simulink model "bus_roadtest_v3"  (R2018a)
settings: Solver=ode3  StartTime=0.0  StopTime=inf  FixedStep=0.01  RelTol=1e-3  EnableMultiTasking=on
PostLoadFcn:
  | , if any(exist('dsrtsu_mdlpostloadfcn', 'file') == [2, 3, 6]), try dsrtsu_mdlpostloadfcn('Execute', bdroot); catch fprintf('Error in PostLoadFcn (dsrtsu_mdlpostloadfcn) for model "%s":\n %s\n', bdroot, lasterr); end, end,
InitFcn:
  | bus_roadtest_v3_initial
values from neighbouring files (symbols this model uses):
  ay_max = 2    [Ini.m]
  delta_t = 0.01    [Ini.m]
  end_left_pass = 1    [Ini.m]
  end_right_pass = 0    [Ini.m]
  finish_node_id = length(Map_data(:,1))    [Ini.m]
  forward_length = 15    [Ini.m]
  gamma = sqrt(N_xaug+lambda)    [bus_roadtest_v3_initial.m]
  k_safe = 1    [Ini.m]
  nodes = nodes(1:index_node,:)    [Ini.m]
  rmin = 10    [Ini.m]
  segments = zeros(length(xy_ends_Pos(:,1)),3)    [Ini.m]
  start_node_id = 1    [Ini.m]
  Ts = 0.01    [bus_roadtest_v3_initial.m]
  Veh_CG = [0.5, 0.2]    [Ini.m]
  Veh_size = [1.99986,6.09558]    [Ini.m]
  vmax = 6    [Ini.m]
  weight = [weight_0,weight_0_cov,weight_i]    [bus_roadtest_v3_initial.m]
undefined symbols (not defined in the file or in its folder): Brake_table, DiscIntNeverNeededParam, Map_data, R, REF_GPS_RFS, Steer_gain_table, T
libraries: rtican x71, simulink x26, rti1401lib_adc_type4 x8, rti1401lib_dio_type4 x1
(part 16 of 18)

== matlab function bus_roadtest_v3/Positioning_module/ITRI_MM/UKF_Only/SLAM_UKF_MM ==
  data: seg_id_near output; Map_data input; dist_op output; Position_X input; op_distance output; Oi_near output; num_lane_direction output; Postion_Y input; Position_H input; seg_heading output; seg_LaneWidth output
function [seg_id_near,dist_op,op_distance,Oi_near,num_lane_direction,seg_heading,seg_LaneWidth]= fcn(Map_data,Position_X,Postion_Y,Position_H)

%%% Map_data=[Seg_XY SLOPE_SEG SHIFT_SEG Heading_X LENGTH_SEG]; nx8
XY_ID=Map_data(:,1);
XY_INI=Map_data(:,2:3);
XY_END=Map_data(:,4:5);
SLOPE_SEG=Map_data(:,6);
SHIFT_SEG=Map_data(:,7);
HEADING_DIFFERENCE_VEH_ROAD = 45*pi/180;
DIST_THREAD_5 = 4;

m=length(XY_ID);
oi_xy=zeros(m,2);
dist_op=zeros(m,1);
for i =1:m
    if SLOPE_SEG(i) == inf
        oi_xy(i,1) = XY_INI(i,1); % x position of the projection point on this segment
        oi_xy(i,2) = Postion_Y;
    elseif SLOPE_SEG(i)==0
        oi_xy(i,1) = Position_X;
        oi_xy(i,2) = XY_INI(i,2);
    else
        a_j = -1/SLOPE_SEG(i);
        b_j = Postion_Y - a_j*Position_X;
        oi_xy(i,1) = (b_j-SHIFT_SEG(i))/(SLOPE_SEG(i)-a_j); % x position of the i-th projection point
        oi_xy(i,2) = (SLOPE_SEG(i)*b_j - a_j*SHIFT_SEG(i))/(SLOPE_SEG(i)-a_j); % y position of the i-th projection point 
    end          
end

for i = 1:length(oi_xy(:,1))
    dist_op(i,1)=sqrt((oi_xy(i,1)-Position_X)^2+(oi_xy(i,2)-Postion_Y)^2);     
end

[seg_id_near,op_distance,oi_near,note,seg_direction,head_err,num_lane_direction,seg_heading] = MM(Position_H*180/pi,[Position_X;Postion_Y],oi_xy,dist_op,Map_data,HEADING_DIFFERENCE_VEH_ROAD,DIST_THREAD_5);
Oi_near=oi_near';
[~,seg_id_ind] = max(XY_ID == seg_id_near);
seg_LaneWidth = Map_data(seg_id_ind,11);
seg_Curvature = Map_data(seg_id_ind,14);

%% MM function
function [seg_id_near,op_distance,oi_near,note,seg_direction,head_err,num_lane_direction,seg_heading] = MM(heading,X_pos,oi_xy,dist_op,Map_data,HEADING_DIFFERENCE_VEH_ROAD,DIST_THREAD_5)
note=0;
seg_id_near=double(0);
op_distance=0;
oi_near=zeros(1,2);
end_pt=zeros(1,2);
seg_direction=0;
[dist_sort,index] = sort(dist_op);
index=[index,zeros(length(index),1)];

xy_ini = Map_data(:,2:3);
xy_end = Map_data(:,4:5);
SLOPE_SEG = Map_data(:,6);
seg_id = Map_data(:,1);
LENGTH_SEG = Map_data(:,9);
SEG_GPS_HEAD = Map_data(:,8);
SEG_GPS_HEAD=[seg_id SEG_GPS_HEAD];

%%    Map Matching

for j = 1:length(xy_ini(:,1));
    i = index(j,1);
    dis_temp1 = sqrt((xy_ini(i,1)-oi_xy(i,1))^2+(xy_ini(i,2)-oi_xy(i,2))^2);
    dis_temp2 = sqrt((xy_end(i,1)-oi_xy(i,1))^2+(xy_end(i,2)-oi_xy(i,2))^2);
 
    if (dis_temp1 <= LENGTH_SEG(i)&& dis_temp2 <= LENGTH_SEG(i));
        index(j,2) = 1; %oi_xy lies in between xy_ini and xy_end
    else index(j,2) = 0;
    end
end

%"possible_seg" contains the sequence of possible segment index
ind_temp = find(index(1:end,2)==1);
% ind_temp=ind_temp(1);
if isempty(ind_temp);
   note = 1;  % 1: the projection point is not between two segment ends for any road segment;
              % search nearest segment by finding the nearest segment end!             
   %compare distances between ends and X_pos!     
    dist_ini = rel_dist_xy(X_pos,xy_ini);
    dist_end = rel_dist_xy(X_pos,xy_end);
  
    [min_dis_ini,junk1] = min(dist_ini);   %-------------------------------------------------哪來的junk 1 &2 ?
    [min_dis_end,junk2] = min(dist_end);
    if min_dis_ini<= min_dis_end; %X_pos is closer to the end
       possible_seg = junk1; %index
       end_pt = xy_ini(junk1,1:end);
    else 
       possible_seg = junk2; %index
       end_pt = xy_end(junk2,1:end);
    end

    seg_id_near = seg_id(possible_seg);
    
    op_distance = dist_op(possible_seg);
    oi_near = oi_xy(possible_seg,1:2);
    if possible_seg>1 && possible_seg<length(seg_id)
    op_distance_n=rel_dist_xy(X_pos,oi_near);
    min_ini_pos=rel_dist_xy(X_pos,xy_ini(possible_seg,:));
    min_end_pos=rel_dist_xy(X_pos,xy_end(possible_seg,:));
    if op_distance_n<min_ini_pos && op_distance_n<min_end_pos
        note = 0;
    else
        note = 1;
    end
    else
        op_distance_n=rel_dist_xy(X_pos,oi_near);
        min_ini_pos=rel_dist_xy(X_pos,xy_ini(possible_seg,:));
        min_end_pos=rel_dist_xy(X_pos,xy_end(possible_seg,:));
    end
    
%    seg_direction = Get_Seg_Heading(seg_id_near,heading);
%    %%%不用老師程式--
    [~,temp_ind] = max(SEG_GPS_HEAD(:,1) == seg_id_near);
    head_err = abs(heading-SEG_GPS_HEAD(temp_ind(1),2)); 
    if head_err <= HEADING_DIFFERENCE_VEH_ROAD
    seg_direction = 1; %1= along slope, 2:adverse
    elseif head_err>=HEADING_DIFFERENCE_VEH_ROAD && head_err<=90
    seg_direction = 0; %unknown
    else
    seg_direction = 2;
    end
%     %%%不用老師程式--
 elseif length(ind_temp(1)) ==1; %only 
%      find one segment candidate
       note = 0; % 0: the projection point lies between two ends of each segment    
       possible_seg = index(ind_temp(1),1);
       seg_id_near = seg_id(possible_seg);
       op_distance = dist_op(possible_seg);
       oi_near = oi_xy(possible_seg,1:2);
       end_pt = [0,0]; % temp./unused nominal values
%      seg_direction = Get_Seg_Heading(seg_id_near,heading); %get road segment heading direction

        [~,temp_ind] = max(SEG_GPS_HEAD(:,1) == seg_id_near);
        head_err = abs(heading-SEG_GPS_HEAD(temp_ind(1),2)); 
       if head_err <= HEADING_DIFFERENCE_VEH_ROAD;
            seg_direction = 1; %1= along slope, 2:adverse
       elseif head_err>=HEADING_DIFFERENCE_VEH_ROAD && head_err<=90
            seg_direction = 0; %unknown
       else
            seg_direction = 2;
       end
       %Now compare the distances between X_pos and all segment ends with
       %op_distance. If find closer node, may discard previous found segment.
       
       dist_ini = rel_dist_xy(X_pos,xy_ini);
       dist_end = rel_dist_xy(X_pos,xy_end);
           %dis_min = min(dist_ini,dist_end);
           %dis_min_val = min(dis_min);
           %temp_a = find(dis_min == dis_min_val); % diff, segments may have the same node!
       [min_dis_ini,junk1] = min(dist_ini);
       [min_dis_end,junk2] = min(dist_end);
       dis_min_val = min(min_dis_ini,min_dis_end);
       
    if dis_min_val < op_distance;%min(op_distance); %X_pos is closer to one of the segment ends than its project point         
       note = 2; %Change the "note" value! 
                 %special case: the found projection pt. (oi_near) lie(s) between two ends 
                 %of one segment, but the associated segments may not
                 %the nearest road segments.          
       %search the nearest node of road segments. 
        if min_dis_ini<= min_dis_end;
           temp_a = junk1;
           end_pt = xy_ini(junk1,1:end);
        else 
           temp_a = junk2;
           end_pt = xy_end(junk2,1:end);
        end
       
        
        if length(temp_a)>1; %multiple segment case
            
           seg_head_pos = SEG_GPS_HEAD(temp_a,2); %road segment heading in the positive slope direction
%            seg_head_neg = SEG_GPS_HEAD(temp_a,3);
           
           %find smallest heading discrepancy in positive slope direction
           [junk1,ind_pos] = min(abs(heading - seg_head_pos(1:end)));
               
           %find smallest heading discrepancy in negative/adverse slope direction
%            [junk2,ind_neg] = min(abs(angle_convert(heading - seg_head_neg(1:end))));
           
           %compare two smallest heading erros of two adverse directions
 
              ind = temp_a(ind_pos);
              seg_id_near = seg_id(ind);
              op_distance = dist_op(ind);
              oi_near = oi_xy(ind,1:2);
              [~,temp_ind] = max(SEG_GPS_HEAD(:,1) == seg_id_near);
              head_err = abs(heading-SEG_GPS_HEAD(temp_ind(1),2)); 

              if head_err <= HEADING_DIFFERENCE_VEH_ROAD;
                    seg_direction = 1; %1= along slope, 2:adverse
              elseif head_err>=HEADING_DIFFERENCE_VEH_ROAD && head_err<=90
                    seg_direction = 0; %unknown
              else
                    seg_direction = 2;
              end
       
        else %single segment case
              [~,temp_ind] = max(SEG_GPS_HEAD(:,1) == seg_id_near);
              head_err = abs(heading-SEG_GPS_HEAD(temp_ind(1),2)); 

              if head_err <= HEADING_DIFFERENCE_VEH_ROAD;
                    seg_direction = 1; %1= along slope, 2:adverse
              elseif head_err>=HEADING_DIFFERENCE_VEH_ROAD && head_err<=90
                    seg_direction = 0; %unknown
              else
                    seg_direction = 2;
              end
                 seg_id_near = seg_id(temp_a);
                 op_distance = dist_op(temp_a);
                 oi_near = oi_xy(temp_a,1:2);
        end
    end
 else %multiple segment candidates
       note = 0; % 0: the projection point lies between two ends of each segment          
       cand_seg = index(ind_temp(1),1);
       %cand_id = seg_id(cand_seg(1:2)); % only check the first two colsest segment candidate
       cand_op_dist = dist_op(cand_seg(1:2));
       
       %find road heading for the first two candidates
        head_pos = SEG_GPS_HEAD(cand_seg(1:2),2);

       %first candidate
        err_1 =  abs(heading - head_pos(1));
        %temp = [head_pos(1),head_neg(1)];
        %cand_head(1) = temp(ii);
        %clear ii;
       %second candidate
        err_2 = abs(heading - head_pos(2));
        %temp = [head_pos(2),head_neg(2)];
        %cand_head(2) = temp(ii);
        %clear ii;
        
       %compare two heading errors
        if err_1<= err_2 && err_1< HEADING_DIFFERENCE_VEH_ROAD; % HEADING_DIFFERENCE_VEH_ROAD = 45/180*pi
           possible_seg =  cand_seg(1);
           seg_direction = 1;
        elseif err_2< err_1 && ((cand_op_dist(2)-cand_op_dist(1))< DIST_THREAD_5); %DIST_THREAD_5 = 9 m
           possible_seg = cand_seg(2); 
           seg_direction = 2;
        else
           possible_seg = cand_seg(1);
           seg_direction = 1;
        end
        
       clear err_1 err_2 cand_op_dist cand_seg head_pos head_neg direction_1 direction_2;
       %possible_seg = index(ind_temp,1);       
       seg_id_near = seg_id(possible_seg);
       op_distance = dist_op(possible_seg);
       oi_near = oi_xy(possible_seg,1:2);
       end_pt = [0,0]; % temp./unused nominal values
        
       %Now compare the distances between X_pos and all segment ends with
       %above op_distance.
       %compute distances between X_pos and all segment ends
       dist_ini = rel_dist_xy(X_pos,xy_ini);
       dist_end = rel_dist_xy(X_pos,xy_end);
           %dis_min = min(dist_ini,dist_end);
           %dis_min_val = min(dis_min);
           %temp_a = find(dis_min == dis_min_val); % diff, segments may have the same node!
       [min_dis_ini,junk1] = min(dist_ini);
       [min_dis_end,junk2] = min(dist_end);
       dis_min_val = min(min_dis_ini,min_dis_end); 
       
    if dis_min_val < op_distance; %min(op_distance); %X_pos is closer to one of the segment ends than its project point         
       note = 2; %Change the note value! 
                 %special case: the found projection pt. (oi_near) lie(s) between two ends 
                 %of one segment, but the associated segments may not be
                 %the nearest road segments.          
       %search the nearest node of road segments. 
        if min_dis_ini<= min_dis_end;
           temp_a = junk1;
           end_pt = xy_ini(junk1,1:2);
        else 
           temp_a = junk2;
           end_pt = xy_end(junk2,1:2);
        end
        clear junk1 junk2;
        
        if length(temp_a)>1; %multiple segment case, then compare heading with road segment heading
          
           seg_head_pos = SEG_GPS_HEAD(temp_a,2);
           [junk1,ind_pos] = min(abs(heading - seg_head_pos(1:end)));


              ind = temp_a(ind_pos);
              seg_id_near = seg_id(ind);
              op_distance = dist_op(ind);
              oi_near = oi_xy(ind,1:2);

              [~,temp_ind] = max(SEG_GPS_HEAD(:,1) == seg_id_near);
              head_err = abs(heading-SEG_GPS_HEAD(temp_ind(1),2)); 

              if head_err <= HEADING_DIFFERENCE_VEH_ROAD;
                    seg_direction = 1; %1= along slope, 2:adverse
              elseif head_err>=HEADING_DIFFERENCE_VEH_ROAD && head_err<=90
                    seg_direction = 0; %unknown
              else
                    seg_direction = 2;
              end

       
        else %determine road direction is positive or negative slope direction

             seg_id_near = seg_id(temp_a);
             op_distance = dist_op(temp_a);
             oi_near = oi_xy(temp_a,1:2);
             [~,temp_ind] = max(SEG_GPS_HEAD(:,1) == seg_id_near);
              head_err = abs(heading-SEG_GPS_HEAD(temp_ind(1),2)); 

              if head_err <= HEADING_DIFFERENCE_VEH_ROAD;
                    seg_direction = 1; %1= along slope, 2:adverse
              elseif head_err>=HEADING_DIFFERENCE_VEH_ROAD && head_err<=90
                    seg_direction = 0; %unknown
              else
                    seg_direction = 2;
              end

        end
    end
           
end
%% check projection distance positive or negative Y=AX+B ;AX+B-Y>0 or AX+B-Y<0
Heading_X_rad = Map_data(:,8).*pi./180;
[~,temp_ind] = max(seg_id(:,1) == seg_id_near);
A=SLOPE_SEG(temp_ind);
B=oi_near(2)-A*oi_near(1);
if A < 0
    C=-A*X_pos(1)-B+X_pos(2);
    if Heading_X_rad(temp_ind) > 3*pi/2 && Heading_X_rad(temp_ind) < 2*pi
        C = C;
    else
        C = -C;
    end
elseif A == 0
    if oi_near(2)<X_pos(2)
        C=-1;
    else
        C=1;
    end
else
    C=A*X_pos(1)+B-X_pos(2);
    if Heading_X_rad(temp_ind) > pi && Heading_X_rad(temp_ind) < 3*pi/2
        C = C;
    else
        C = -C;
    end
end
if C<0 
    d=1;
elseif C==0
    d=1;
else
    d=-1;
end
num_lane_direction=[A;B;C;d];
seg_heading = Heading_X_rad(temp_ind);
%% rel_dist
function dist = rel_dist_xy(ref_xy,pt_xy)
% This function computes relative distances between given reference point, ref_xy, and positions, p_xy. 
% ref_xy = [x0,y0];
% pt_xy = [x,y];

temp = (pt_xy(:,1)-ref_xy(1)).^2 + (pt_xy(:,2)-ref_xy(2)).^2;
dist = temp.^0.5;

== matlab function bus_roadtest_v3/Positioning_module/ITRI_MM/UKF_Only/SLAM_UKF ==
  data: Q input; R input; X output; X_AUG input; X_state input; IMU_Sensor input; Sensor_dt input; SLAM_update input; weighting input; P output; K output; x_aug output; d_GC input
function [X,P,K,x_aug] = fcn(Q,R,X_AUG,X_state,IMU_Sensor,Sensor_dt,SLAM_update,weighting,d_GC)
%#codegen

%% parameters setup

%%% X_State=[X,Y,Heading]
x_aug=X_AUG(:,1:11);
vx=IMU_Sensor(1)*1;
wz=IMU_Sensor(2);
Grade=IMU_Sensor(3);
dt=Sensor_dt;
weight_0=weighting(1);
weight_0_cov=weighting(2);
weight_i=weighting(3);
X=zeros(5,1);
N=5;

%%
%%% model 1 : slope detection
    x_aug(1,:) = x_aug(1,:) + (dt*x_aug(5,:)).*cos(x_aug(3,:)) + dt.*wz*d_GC*cos(x_aug(3,:)+pi/2); %north
    x_aug(2,:) = x_aug(2,:) + (dt*x_aug(5,:)).*sin(x_aug(3,:)) + dt.*wz*d_GC*sin(x_aug(3,:)+pi/2);%east
    x_aug(3,:) = x_aug(3,:) + (dt.*x_aug(4,:));                  %heading (radian)
    x_aug(4,:) = x_aug(4,:);
    x_aug(5,:) = x_aug(5,:);
    

 %% state process

X(1,1) = x_aug(1,1)*weight_0 + sum(x_aug(1,2:end))*weight_i;
X(2,1) = x_aug(2,1)*weight_0 + sum(x_aug(2,2:end))*weight_i;
X(3,1) = x_aug(3,1)*weight_0 + sum(x_aug(3,2:end))*weight_i;
X(4,1) = x_aug(4,1)*weight_0 + sum(x_aug(4,2:end))*weight_i;
X(5,1) = x_aug(5,1)*weight_0 + sum(x_aug(5,2:end))*weight_i;
% X = X*10^6;

    P = weight_0_cov.*((x_aug(1:5,1)-X(1:5,1))*(x_aug(1:5,1)-X(1:5,1))');

for i = 2:(2*N+1)
    
    P = P + weight_i.*((x_aug(1:5,i)-X(1:5,1))*(x_aug(1:5,i)-X(1:5,1))');

end
% P = P*10^6;

P = P + Q;

if X(3,1) < 0
    X(3,1) = X(3,1) + 2*pi;
elseif X(3,1) >= 2*pi
    X(3,1) = X(3,1) - 2*pi;
else
    X(3,1) = X(3,1);
end
%% kalman filter
if SLAM_update >0 %close-loop
    
 
        Z = X_state;

        Z_e = X; %=H*X; % observation estimate using a-priori state estimate
   %K = P*H'*inv(H*P*H'+R); % Kalman gain
        K = P*inv(P+R); %H = eye(3) %K = P*inv(P+R)
   %X = X + K*(Z - Z_e); % a-posteriori state estimate
        dZ = Z - Z_e;
        X = X + K*dZ; % a-posteriori state estimate
   
   %P = (eye(3) - K*H)*P;
  
   
        P = (eye(5) - K)*P;

        
else %open loop
        
        K = zeros(5,5);
        Z = X_state([4,5]); 
        Z_e = X([4,5]); %=H*X; % observation estimate using a-priori state estimate
   %K = P*H'*inv(H*P*H'+R); % Kalman gain
        K1 = P([4,5],([4,5]))*inv(P([4,5],([4,5]))+R([4,5],([4,5]))); %H = eye(3)
   %X = X + K*(Z - Z_e); % a-posteriori state estimate
        dZ = Z - Z_e;
        X([4,5]) = X([4,5]) + K1*dZ; % a-posteriori state estimate
   
   %P = (eye(3) - K*H)*P;
    
        P([4,5],([4,5])) = (eye(2) - K1)*P([4,5],([4,5]));
end


function dist = rel_dist_xy(ref_xy,pt_xy)
% This function computes relative distances between given reference point, ref_xy, and positions, p_xy. 
% ref_xy = [x0,y0];
% pt_xy = [x,y];

temp = (pt_xy(:,1)-ref_xy(1)).^2 + (pt_xy(:,2)-ref_xy(2)).^2;
dist = temp.^0.5;

== matlab function bus_roadtest_v3/Positioning_module/ITRI_MM/UKF_Only/SLAM_Check ==
  data: SLAM_fault input; SLAM_X input; SLAM_update output; SLAM_Y input; SLAM_Heading input; SLAM_Counter input; IMU_Sensor input; X_UKF input; SLAM_FS input; Q_last_i input; R_last_i input; Last_SLAM_In input; X_state output; SLAM_FaultFlag output; Q_last_o output; R_last_o output; Last_SLAM_Out output; count_i input; count_o output; dist_SLAMlastUKFSLAM output; SLAM_FaultFlag_case output
function [SLAM_update,X_state,SLAM_FaultFlag,Q_last_o,R_last_o,Last_SLAM_Out,count_o,dist_SLAMlastUKFSLAM,SLAM_FaultFlag_case] = fcn(SLAM_fault,SLAM_X,SLAM_Y,SLAM_Heading,SLAM_Counter,IMU_Sensor,X_UKF,SLAM_FS,Q_last_i,R_last_i,Last_SLAM_In,count_i)

Last_X=Last_SLAM_In(1);
Last_Y=Last_SLAM_In(2);
Last_Heading = Last_SLAM_In(3);
Last_Counter = Last_SLAM_In(4);

Sensor_Velocity = IMU_Sensor(1);
Sensor_Yawrate=IMU_Sensor(2);
Sensor_Grade=IMU_Sensor(3);

SLAM_FaultFlag = 0;
SLAM_update = 0;

if SLAM_Counter ~= Last_Counter
    SLAM_update = 1;
    count_o = 0;
else
    count_o = count_i + 1;
end

if SLAM_fault == 1
    SLAM_update = 0;
end

SLAM_FaultFlag_case = 0;
dist_SLAMlastUKFSLAM = sqrt((SLAM_X-X_UKF(1))^2 + (SLAM_Y-X_UKF(2))^2); %跟上一刻估測值差異
dist_SLAMlastSLAM =  sqrt((SLAM_X-Last_X)^2 + (SLAM_Y-Last_Y)^2); %跟上一刻量測值差異
Heading_diff = abs(SLAM_Heading-Last_Heading);
if Heading_diff > pi
    Heading_diff = 2*pi - Heading_diff;
end
if Sensor_Velocity < 0.01
    if SLAM_fault == 1 || count_o > 100 || dist_SLAMlastUKFSLAM > 0.1
        SLAM_FaultFlag = 1;
        SLAM_FaultFlag_case = 1;
    end
    if SLAM_update > 0 && dist_SLAMlastSLAM > 0.1
        SLAM_FaultFlag = 1;
        SLAM_FaultFlag_case = 2;
    end
    if SLAM_update > 0 && Heading_diff > 20*pi/180
        SLAM_FaultFlag = 1;
        SLAM_FaultFlag_case = 3;
    end
else
    if SLAM_fault == 1 || count_o > 200 || dist_SLAMlastUKFSLAM > 5
        SLAM_FaultFlag = 1;
        SLAM_FaultFlag_case = 4;
    end
end

if abs(SLAM_Heading - X_UKF(3)) > 5.5
    H_ACC = 100;
else
    H_ACC = 0.1;
end

if SLAM_update == 0
    SLAM_X_out = Last_X;
    SLAM_Y_out = Last_Y;
    SLAM_Heading_out = Last_Heading;
    Q = Q_last_i;
    R = R_last_i;
else
    SLAM_X_out = SLAM_X;
    SLAM_Y_out = SLAM_Y;
    SLAM_Heading_out = SLAM_Heading;
    Q = diag([0.00025,0.00025,0.0000001,0.00001,0.0001]);
    R = diag([(0.01)^2,(0.01)^2,H_ACC,0.1,0.0001]);
end

Q_last_o = Q;
R_last_o = R;
SLAM_Counter_out = SLAM_Counter;

Last_SLAM_Out = [SLAM_X_out;SLAM_Y_out;SLAM_Heading_out;SLAM_Counter_out];
X_state = [SLAM_X_out,SLAM_Y_out,SLAM_Heading_out,Sensor_Yawrate,Sensor_Velocity]';

== matlab function bus_roadtest_v3/Speed_profile/Auto & Check/Auto_Door ==
  settings: updateMethod=DISCRETE
  data: Static_flag input; Auto_Door output; Stop_Check input; Door_count output
function [Auto_Door, Door_count] = fcn(Static_flag,Stop_Check)
persistent counting Stop_state
if isempty(counting)
    counting = 0;
    Stop_state = 0;
end
Auto_Door = 0;

if Stop_Check ==1
    Stop_state = 1;
end
if Stop_state==1 && Static_flag==1
    counting = counting+1;
end
if counting>300
    Auto_Door=1;
    Stop_state = 0;
    counting = 0;
end
Door_count = counting;

== matlab function bus_roadtest_v3/Data_RX/X-by-wire/Steer/CAN_timeout_checker ==
  data: RX_sig input; timeout output
function timeout = fcn(RX_sig)
persistent counter
if isempty(counter)
    counter = 0;
end

if (RX_sig == 0)
    counter = counter +1;
else
    counter = 0;
end

if counter >= 80
    timeout = 1;
else
    timeout = 0;
end

== matlab function bus_roadtest_v3/Target_planner/Path_Output ==
  settings: updateMethod=DISCRETE  sampleTime=0.01
  data: Vehicle_state input; Path_LV output; Path_x input; Path_y input
function Path_LV  = TargetDecision(Vehicle_state,Path_x,Path_y)
%% projection Path to LiDAR view
x = Vehicle_state(1,1);
y = Vehicle_state(2,1);
heading = Vehicle_state(3,1);

Path_LV = zeros(2,6);
% for i =1:6
%     j = i + 1;
%     rotate_ang_path = (heading-pi/2);
%     Path_LV(1:2,i) = [cos(rotate_ang_path),sin(rotate_ang_path);-sin(rotate_ang_path),cos(rotate_ang_path)]*[Path_x(j)-x;Path_y(j)-y];
% end

== matlab function bus_roadtest_v3/Flag_management/Fault detection/Fault detection(Control)/Brake fault detection/MATLAB Function2 ==
  data: u input; y output
function y = my_average(u) %# codegen
persistent i buf bufSum;
if isempty(buf)
    buf = zeros(1,300); %averaging steps
    bufSum = 0;
    i = 1;
end
bufSum = bufSum - buf(i);
buf(i) = u;
bufSum = bufSum + u;
i = i + 1;
if i > numel(buf)
    i = 1;
end
y = bufSum / numel(buf);

== matlab function bus_roadtest_v3/Flag_management/Fault detection/Fault detection(Control)/Steer fault detection/MATLAB Function4 ==
  settings: updateMethod=DISCRETE
  data: u input; y output
function y = my_average(u) %# codegen
persistent i buf bufSum;
if isempty(buf)
    buf = zeros(1,200); %averaging steps
    bufSum = 0;
    i = 1;
end
bufSum = bufSum - buf(i);
buf(i) = u;
bufSum = bufSum + u;
i = i + 1;
if i > numel(buf)
    i = 1;
end
y = bufSum / numel(buf);

== matlab function bus_roadtest_v3/Flag_management/Fault detection/Fault detection(Control)/Steer fault detection/MATLAB Function5 ==
  settings: updateMethod=DISCRETE
  data: u input; y output
function y = my_average(u) %# codegen
persistent i buf bufSum;
if isempty(buf)
    buf = zeros(1,50); %averaging steps
    bufSum = 0;
    i = 1;
end
bufSum = bufSum - buf(i);
buf(i) = u;
bufSum = bufSum + u;
i = i + 1;
if i > numel(buf)
    i = 1;
end
y = bufSum / numel(buf);

== matlab function bus_roadtest_v3/Flag_management/Fault detection/Fault detection(Control)/Speed fault detection/MATLAB Function6 ==
  settings: updateMethod=DISCRETE
  data: u input; y output
function y = my_average(u) %# codegen
persistent i buf bufSum;
if isempty(buf)
    buf = zeros(1,500); %averaging steps
    bufSum = 0;
    i = 1;
end
bufSum = bufSum - buf(i);
buf(i) = u;
bufSum = bufSum + u;
i = i + 1;
if i > numel(buf)
    i = 1;
end
y = bufSum / numel(buf);

== matlab function bus_roadtest_v3/Flag_management/Fault detection/Fault detection(Control)/Speed fault detection/MATLAB Function7 ==
  settings: updateMethod=DISCRETE
  data: u input; y output
function y = my_average(u) %# codegen
persistent i buf bufSum;
if isempty(buf)
    buf = zeros(1,50); %averaging steps
    bufSum = 0;
    i = 1;
end
bufSum = bufSum - buf(i);
buf(i) = u;
bufSum = bufSum + u;
i = i + 1;
if i > numel(buf)
    i = 1;
end
y = bufSum / numel(buf);

== matlab function bus_roadtest_v3/Flag_management/Fault detection/Fault detection(Control)/OBU fault detection ==
  data: SPAT input; OBU_fault output; counting output
function [OBU_fault, counting] = fcn(SPAT)

persistent count;
if isempty(count)
    count = 0;
end

count = count +1;
if SPAT == 1
    count = 0;
end
OBU_fault = 0;
if count>300
    OBU_fault = 1;
end
counting = count;

== matlab function bus_roadtest_v3/Flag_management/Fault detection/Fault flags management ==
  data: Fault_minor output; Fault_prime output; Monitor_fault input; OBU_fault input; Speed_fault input; Steer_fault input; Brake_fault input; RSU_fault input; SLAM_fault input
function [Fault_minor, Fault_prime] = fcn(Monitor_fault, OBU_fault, Speed_fault, Steer_fault, Brake_fault,RSU_fault,SLAM_fault)
Fault_prime = max([Monitor_fault, OBU_fault, Speed_fault, Steer_fault, Brake_fault, RSU_fault, SLAM_fault]);
% if Uturn_flag==1
%     Fault_prime = 0;
% end
Fault_minor = 0;

== matlab function bus_roadtest_v3/Flag_management/Button management/Button management ==
  settings: updateMethod=DISCRETE
  data: Drive_start_button input; Drive_stop_button input; Drive_start output; Emergency_button input; Door_state_fb input; Door1_open_button input; Door1_close_button input; Door2_button input; Door_switch_button input; Drive_stop output; Emergency_stop output; Door_cmd output; Auto_Door input
function [Drive_start, Drive_stop, Emergency_stop, Door_cmd] = Button_management(Drive_start_button, Drive_stop_button, Emergency_button, Door_state_fb, Door1_open_button, Door1_close_button, Door2_button, Door_switch_button, Auto_Door)

%For Door control
% Door_switch   0=Operator  1=Passenger
% Door_state    0 = close   1 = open  
%Door_button = [Door_state_fb, Door1_open_button, Door1_close_button, Door2_button, Door_switch_button];

persistent Door_state Time_count;
if isempty(Time_count)
    Door_state = Door_state_fb;
    Time_count = 0;
end 

if Door_switch_button == 0
    if Door1_open_button ==1
        Door_state = 1;
    elseif Door1_close_button ==1
        Door_state = 0;
    end
elseif Door_switch_button == 1
    if  Door2_button ==1 && Time_count >500  % Door can't change twice within 5 second
        if Door_state ==1
            Door_state = 0;
        else
            Door_state = 1;
        end
        Time_count = 0;
    end
    if Door1_open_button ==1
        Door_state = 1;
    elseif Door1_close_button ==1
        Door_state = 0;
    end
end
Time_count = Time_count + 1;
if Auto_Door ==1
    Door_state = 1;
end



Door_cmd = Door_state;
Emergency_stop = Emergency_button; 
Drive_start =Drive_start_button;
Drive_stop = Drive_stop_button;




%%%%%%%%%%%%%%%%%%%%%%%%%%%%%%%%%%%%%%%%%%%%%%%%%%%%%%%%%%%%%%%%%%%%%%%%%%%

== matlab function bus_roadtest_v3/Data_RX/X-by-wire/Brake/CAN_timeout_checker ==
  data: RX_sig input; timeout output
function timeout = fcn(RX_sig)
persistent counter
if isempty(counter)
    counter = 0;
end

if (RX_sig == 0)
    counter = counter +1;
else
    counter = 0;
end

if counter >= 80
    timeout = 1;
else
    timeout = 0;
end

== matlab function bus_roadtest_v3/Data_RX/Control_button/MATLAB Function2 ==
  settings: updateMethod=DISCRETE
  data: u input; y output; yy output
function [y,yy]= fcn(u)
%#codegen
persistent y2 y1 ;
if isempty(y2)
    y2 = 0;
    y1 = 0;
end 
if u ==1
    y2 = 1;
end
yy = y2;
y = y1;

== matlab function bus_roadtest_v3/Data_RX/X-by-wire/Brake/CAN_timeout_checker1 ==
  data: RX_sig input; timeout output
function timeout = fcn(RX_sig)
persistent counter
if isempty(counter)
    counter = 0;
end

if (RX_sig == 0)
    counter = counter +1;
else
    counter = 0;
end

if counter >= 80
    timeout = 1;
else
    timeout = 0;
end

== matlab function bus_roadtest_v3/Data_RX/X-by-wire/Throttle/CAN_timeout_checker ==
  data: RX_sig input; timeout output
function timeout = fcn(RX_sig)
persistent counter
if isempty(counter)
    counter = 0;
end

if (RX_sig == 0)
    counter = counter +1;
else
    counter = 0;
end

if counter >= 80
    timeout = 1;
else
    timeout = 0;
end

== matlab function bus_roadtest_v3/Data_RX/OBU/Light_state_DSRC ==
  settings: updateMethod=DISCRETE
  data: SLAM_seg_id_near input; phase_01 input; Light_info_out output; phase_02 input; phase_03 input; phase_04 input; phase_05 input; phase_06 input; phase_07 input; phase_08 input; RT_01 input; RT_02 input; RT_03 input; RT_04 input; RT_05 input; red output; left output; last_phase input
function [Light_info_out,red,left]     = fcn(SLAM_seg_id_near,phase_01,phase_02,phase_03,phase_04,phase_05,phase_06,phase_07,phase_08, RT_01, RT_02, RT_03, RT_04,RT_05,last_phase)

% output light info 0=no message, 1=red, 2=green,3=yellow

persistent Light_info;
if isempty(Light_info)
    Light_info = 0;
end 
phase01 = de2bi(phase_01);
phase02 = de2bi(phase_02);
if phase_02<128
    phase02(8)=0;
end
phase03 = de2bi(phase_03);
phase04 = de2bi(phase_04);
phase05 = de2bi(phase_05);
phase06 = de2bi(phase_06);
phase07 = de2bi(phase_07);
phase08 = de2bi(phase_08);

if SLAM_seg_id_near>=999 && SLAM_seg_id_near<134
    if phase01(6)==1  || phase01(4)==1
        Light_info =2;
    else
        Light_info =1;
    end
% elseif SLAM_seg_id_near>=134 && SLAM_seg_id_near<154
% || (phase02(8)==1&&last_phase==0&&RT_02<10)
elseif SLAM_seg_id_near>=134 && SLAM_seg_id_near<154
     if (phase02(6)==1&&RT_02>2)  || (phase02(5)==1&&RT_02>2) || (phase02(8)==1&&last_phase==0&&RT_02<16)
        Light_info =2;
    else
        Light_info =1;
    end
elseif SLAM_seg_id_near>=218 && SLAM_seg_id_near<238
    if (phase05(6)==1&&RT_05>3)  || phase05(4)==1
        Light_info =2;
    else
        Light_info =1;
    end
elseif SLAM_seg_id_near>=238 && SLAM_seg_id_near<252
    if (phase04(6)==1&&RT_04>3)  || phase04(4)==1
        Light_info =2;
    else
        Light_info =1;
    end
elseif SLAM_seg_id_near>=252 && SLAM_seg_id_near<267
    if (phase03(6)==1&&RT_03>3)  || phase03(5)==1
        Light_info =2;
    else
        Light_info =1;
    end
elseif SLAM_seg_id_near>=309 && SLAM_seg_id_near<329
    if phase08(6)==1  || phase08(5)==1
        Light_info =2;
    else
        Light_info =1;
    end
else
    Light_info =0;
end

Light_info_out = Light_info;
red = phase02(8);
left = phase02(5);

== matlab function bus_roadtest_v3/Data_RX/X-by-wire/Input_speed/MATLAB Function ==
  settings: updateMethod=DISCRETE
  data: Speed_raw input; Speed_mps output; Rate_limit input
function Speed_mps = Spike_filter(Speed_raw,Rate_limit)

persistent Speed_mps_last
if isempty(Speed_mps_last)
    Speed_mps_last = 0;
end 

if abs(Speed_raw - Speed_mps_last) > Rate_limit
    Speed_mps = Speed_mps_last + sign(Speed_raw-Speed_mps_last) * Rate_limit;
else
    Speed_mps = Speed_raw;
end

Speed_mps_last = Speed_mps;

== matlab function bus_roadtest_v3/Data_RX/Xavier/Filter1/MATLAB Function ==
  data: GF input; GF_filtered output; GF_last input
function GF_filtered  = fcn(GF,GF_last)
persistent count
if isempty(count)
    count = 0;
end

if (GF_last-GF) > 200 && count<20
    GF_filtered = GF_last;
    count = count+1;
else
    GF_filtered = GF;
    count = 0;
end

== matlab function bus_roadtest_v3/Data_RX/Xavier/Filter2/MATLAB Function ==
  data: GF input; GF_filtered output; GF_last input
function GF_filtered  = fcn(GF,GF_last)
persistent count
if isempty(count)
    count = 0;
end

if (GF_last-GF) > 200 && count<10
    GF_filtered = GF_last;
    count = count+1;
else
    GF_filtered = GF;
    count = 0;
end

== matlab function bus_roadtest_v3/Data_RX/OBU/Check_New_SBG_and_x_y_coordination ==
  data: x output; y output; SBG_long input; SBG_lat input; SBG_alt input; REF_GPS_RFS input; z output
function [x,y,z] = fcn(SBG_long,SBG_lat,SBG_alt,REF_GPS_RFS)
%#codegen
[x,y,z] = dllh2denu(REF_GPS_RFS,[SBG_long,SBG_lat,SBG_alt]) ;

function [de,dn,du] =dllh2denu(llh0,llh)
%%% approximation version for GPS coordinate transformation from
%%% llh(longitude,latitude,altitude) to [de,dn,du]=(east,north,height) relatitive to a
%%% given reference point,llh0
% REF_GPS_RFS = [122.000000+20.0304416/60, 37.000000+54.8767679/60, 10.2266];  
% REF_GPS_RFS(1) = -REF_GPS_RFS(1); % Longitude: (-):West, (+):East

%%%%%constants
a = 6378137;
b = 6356752.3142;
e2 = 1 - (b/a)^2;
%%%%%% location of reference point in radians
phi = llh0(2)*pi/180;
lam = llh0(1)*pi/180;
h = llh0(3);
%%%%%%location of data points in radians
dphi = llh(:,2)*pi/180 - phi; % LATITUDE
dlam = llh(:,1)*pi/180 -lam;  % LONGITUDE
dh = llh(:,3)-h;  %altitude
%%%%%%% some useful definitions
tmp1 = sqrt(1-e2*sin(phi)^2);
% cl = cos(lam);
% sl = sin(lam);
cp = cos(phi);
sp = sin(phi);
%%%%%% Transformations
de = (a/tmp1+h)*cp*dlam- (a*(1-e2)/(tmp1^3)+h)*sp.*dphi.*dlam+cp.*dlam.*dh;
dn = (a*(1-e2)/tmp1^3+h)*dphi+1.5*cp*sp*a*e2*dphi.^2+sp^2.*dh.*dphi+0.5*sp*cp*(a/tmp1+h)*dlam.^2;
du = dh -0.5*(a-1.5*a*e2*cp^2+0.5*a*e2+h)*dphi.^2-0.5*cp^2*(a/tmp1-h)*dlam.^2;
%denu2 = [de,dn,du];
%%%%%%%%%%%%%%%%%%%%%%%%%%%

== matlab function bus_roadtest_v3/Positioning_module/ITRI_MM/UKF_Only/ENU2SLAM ==
  data: Car_x input; Car_SLAM_x output; Car_y input; Car_z input; R input; T input; Car_SLAM_y output; Car_SLAM_z output
function [Car_SLAM_x,Car_SLAM_y,Car_SLAM_z] = fcn(Car_x,Car_y,Car_z,R,T)
R_1 = R(:,1:3);
R_2 = R(:,4:6);
R_3 = R(:,7:9);
R_4 = R(:,10:12);
R_5 = R(:,13:15);

T_1 = T(:,1);
T_2 = T(:,2);
T_3 = T(:,3);
T_4 = T(:,4);
T_5 = T(:,5);

if Car_x <= 0
    R_final = R_1;
    T_final = T_1;
elseif Car_x > 0 && Car_x <= 100
    R_final = R_2;
    T_final = T_2;
elseif Car_x > 100 && Car_x <= 225
    R_final = R_3;
    T_final = T_3;
elseif Car_x > 225 && Car_x <= 350
    R_final = R_4;
    T_final = T_4;
else
    R_final = R_5;
    T_final = T_5;
end

% R_final = R;
% T_final = T;

Car_SLAM_xyz = R_final*[Car_x;Car_y;Car_z] + T_final ;

Car_SLAM_x = Car_SLAM_xyz(1);
Car_SLAM_y = Car_SLAM_xyz(2);
Car_SLAM_z = Car_SLAM_xyz(3);

== matlab function bus_roadtest_v3/Data_RX/OBU/TrafficLightFilter ==
  data: V2X_Phase input; V2X_Phase_out output; V2X_Remaintime input; SLAM_seg_id_near input; V2X_Remaintime_out output
function [V2X_Phase_out, V2X_Remaintime_out] = fcn(V2X_Phase, V2X_Remaintime,SLAM_seg_id_near)

% if (SLAM_seg_id_near<113 && SLAM_seg_id_near>104)
    V2X_Phase_out = V2X_Phase;
    V2X_Remaintime_out  = V2X_Remaintime;
% else
%     V2X_Phase_out = 0;
%     V2X_Remaintime_out = -1;
% end

== matlab function bus_roadtest_v3/Positioning_module/ITRI_MM/UKF_Only/MATLAB Function1 ==
  data: Map_data input; forward_path output; seg_id_near input; forward_segid output; Map_switch input
function [forward_path,forward_segid] = fcn(Map_data,seg_id_near,Map_switch)

if Map_switch > 0
    if seg_id_near >= 38 && seg_id_near <= 100
        forward_path_ = [Map_data(end,:);Map_data(end,:);Map_data(end,:);Map_data(end,:);Map_data(end,:)];
        [~,seg_start_ind] = max(Map_data(:,1) == seg_id_near);
        if seg_start_ind + 4 <= length(Map_data(:,1))
            seg_end_ind = seg_start_ind + 4;
        else
            seg_end_ind = length(Map_data(:,1));
        end
        index = 0;
        for i = seg_start_ind : seg_end_ind
            index = index + 1;
            forward_path_(index,:) = Map_data(i,:);
        end
        length_Map = length(Map_data(:,1));
        temp = ones((length_Map-5),1)*Map_data(seg_end_ind,:);
        forward_path = [forward_path_;temp];
    else
        forward_path = Map_data;
    end
else
    forward_path = Map_data;
end

forward_segid = forward_path(:,1);

== matlab function bus_roadtest_v3/Target_planner/DangerousArea ==
  data: OB_num input; OBXY input; w_off output; End_x input; End_y input; vehicle_position input; Forward_Static_Path_id input size=length(nodes(:,1)); Static_Path_0 input size=size(Map_data); forward_length input; last_avoidancemode input; avoidancemode output; last_H_x input; last_H_y input; H_x_out output; H_y_out output; count_i input; count_o output
function [w_off,avoidancemode,H_x_out,H_y_out,count_o] = DA(OB_num,OBXY,End_x,End_y,vehicle_position,Forward_Static_Path_id,Static_Path_0,forward_length,last_avoidancemode,last_H_x,last_H_y,count_i)
avoidancemode = last_avoidancemode;
H_x_out = last_H_x;
H_y_out = last_H_y;
flag = 0;

x = vehicle_position(1,1); %vehicle global coordinate
y = vehicle_position(2,1);

Forward_Static_Path_0 = zeros(length(Forward_Static_Path_id),length(Static_Path_0(1,:)));
for i = 1 : length(Forward_Static_Path_id)
    [~,ind] = max(Forward_Static_Path_id(i) == Static_Path_0(:,1));
    Forward_Static_Path_0(i,:) = Static_Path_0(ind,:);
end
for m = 1 : OB_num
    OBXY_m = OBXY(2*m-1:2*m,1:4);
    for j = 1 : length(Forward_Static_Path_id)
        x1 = Forward_Static_Path_0(j,2);
        y1 = Forward_Static_Path_0(j,3);
        x2 = Forward_Static_Path_0(j,4);
        y2 = Forward_Static_Path_0(j,5);
        a = y2-y1;
        b = x1-x2;
        c = -x1*(y2-y1)+y1*(x2-x1);
        D = abs((a*OBXY_m(1,:) + b*OBXY_m(2,:) + c*ones(1,length(OBXY_m(1,:)))))./sqrt(a^2+b^2);
        H_x = (b^2*OBXY_m(1,:)-a*b*OBXY_m(2,:)-a*c)/(a^2+b^2);
        H_y = (-a*b*OBXY_m(1,:)+a^2*OBXY_m(2,:)-b*c)/(a^2+b^2);
        vehicle_x_H = (b^2*x-a*b*y-a*c)/(a^2+b^2);
        vehicle_y_H = (-a*b*x+a^2*y-b*c)/(a^2+b^2);
        xx = [vehicle_x_H,End_x];
        yy = [vehicle_y_H,End_y];
%         if End_x <= max(H_x) && End_x >= min(H_x) && End_y <= max(H_y) && End_y >= min(H_y) && min(D) <= Forward_Static_Path_0(j,11)/2
%             avoidancemode = 1;
%             H_x_out = H_x';
%             H_y_out = H_y';
%             flag = 1;
%             break;
%         elseif max(H_x) <= max(xx) && max(H_x) >= min(xx) && max(H_y) <= max(yy) && max(H_y) >= min(yy) && min(D) <= Forward_Static_Path_0(j,11)/2
%             avoidancemode = 1;
%             H_x_out = H_x';
%             H_y_out = H_y';
%             flag = 1;
%             break;
        if min(H_x) <= max(xx) && max(H_x) >= min(xx) && min(H_y) <= max(yy) && max(H_y) >= min(yy) && min(D) <= Forward_Static_Path_0(j,11)/2
            avoidancemode = 1;
            H_x_out = H_x';
            H_y_out = H_y';
            flag = 1;
            break;
        else
            avoidancemode = last_avoidancemode;
            H_x_out = last_H_x;
            H_y_out = last_H_y;
            flag = 0;
        end
    end
    if flag == 1
        break;
    end
end
% if Path_flag == 0
%     avoidancemode = 0;
% end

if avoidancemode == 1
    if sqrt(min((End_x*ones(4,1)-H_x_out).^2+(End_y*ones(4,1)-H_y_out).^2)) > forward_length + 3
        avoidancemode = 0;
    end
end
if avoidancemode == 1
    count_o = 100;
    w_off = 5;
else
    count_o = count_i - 1;
    if count_o < 0
        count_o = 0;
    end
    w_off = 5*(100-count_o)/100 + 5;
end

== matlab function bus_roadtest_v3/Data_TX/IPC/ENU2SLAM ==
  data: Car_x input; Car_SLAM_x output; Car_y input; Car_z input; R input; T input; Car_SLAM_y output; Car_SLAM_z output
function [Car_SLAM_x,Car_SLAM_y,Car_SLAM_z] = fcn(Car_x,Car_y,Car_z,R,T)

R_1 = R(:,1:3);
R_2 = R(:,4:6);
R_3 = R(:,7:9);
R_4 = R(:,10:12);
R_5 = R(:,13:15);

T_1 = T(:,1);
T_2 = T(:,2);
T_3 = T(:,3);
T_4 = T(:,4);
T_5 = T(:,5);

if Car_x <= 0
    R_final = R_1;
    T_final = T_1;
elseif Car_x > 0 && Car_x <= 100
    R_final = R_2;
    T_final = T_2;
elseif Car_x > 100 && Car_x <= 225
    R_final = R_3;
    T_final = T_3;
elseif Car_x > 225 && Car_x <= 350
    R_final = R_4;
    T_final = T_4;
else
    R_final = R_5;
    T_final = T_5;
end

% R_final = R;
% T_final = T;

Car_SLAM_xyz = R_final*[Car_x;Car_y;Car_z] + T_final ;

Car_SLAM_x = Car_SLAM_xyz(1);
Car_SLAM_y = Car_SLAM_xyz(2);
Car_SLAM_z = Car_SLAM_xyz(3);
